simulink model "simulink_course_proj"  (R2026a)
settings: Solver=VariableStepAuto  StopTime=2
libraries: slpidlib x1
settings Model: Creator=noahhansen  LastModifiedBy=noahhansen

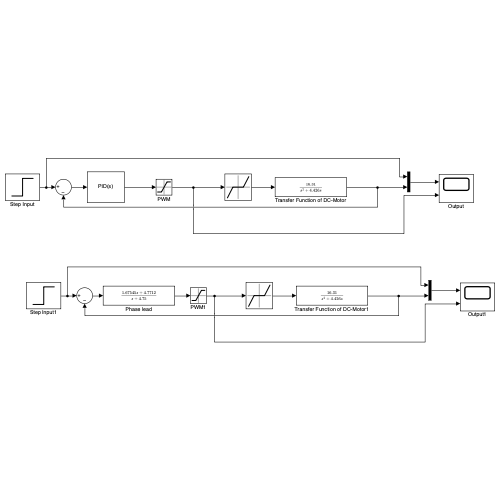
[thumbnail: Simulink's stored preview of the top-level diagram]
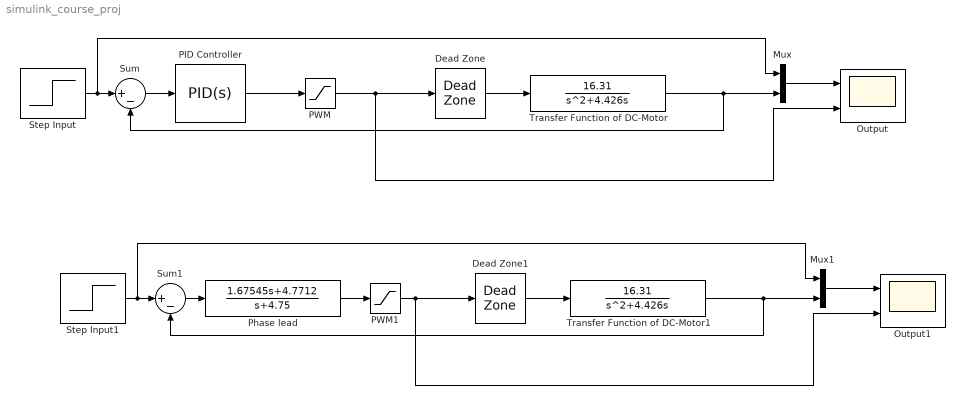
== system simulink_course_proj ==
  Dead Zone : DeadZone  LowerValue=-40  UpperValue=40
  Dead Zone1 : DeadZone  LowerValue=-40  UpperValue=40
  Mux : Mux  Inputs=2
  Mux1 : Mux  Inputs=2
  Output : Scope  NumInputPorts=2
      settings: TimeDisplayOffset=-0.1  ActiveDisplayYMinimum=-2  ActiveDisplayYMaximum=25  YLabel=Angle (degrees)
  Output1 : Scope  NumInputPorts=2
      settings: TimeDisplayOffset=-0.1  ActiveDisplayYMinimum=-10.6993  ActiveDisplayYMaximum=40  YLabel=Angle (degrees)
  PID Controller : slpidlib/PID Controller  Controller=PID  Form=Parallel  TimeDomain=Continuous-time  UseExternalTs=off  SampleTime=-1  IntegratorMethod=Forward Euler  FilterMethod=Forward Euler  ControllerParametersSource=internal  P=29  I=5  UseKiTs=off  D=1.4  UseExternalDerivativeSource=off  N=100  UseFilter=on  TunerSelectOption=Transfer Function Based (PID Tuner App)  InitialConditionSource=internal  InitialConditionForIntegrator=0  InitialConditionForFilter=0  DifferentiatorICPrevScaledInput=0  ExternalReset=none  TrackingMode=off  Kt=1  LimitOutput=off  SatLimitsSource=internal  UpperSaturationLimit=inf  LowerSaturationLimit=-inf  LinearizeAsGain=on  AntiWindupMode=none  Kb=1  LimitIntegrator=off  UpperIntegratorSaturationLimit=inf  LowerIntegratorSaturationLimit=-inf  POutMin=[]  POutMax=[]  IOutMin=[]  IOutMax=[]  DOutMin=[]  DOutMax=[]  NOutMin=[]  NOutMax=[]  SumOutMin=[]  SumOutMax=[]  SaturationOutMin=[]  SaturationOutMax=[]  PParamMin=[]  PParamMax=[]  IParamMin=[]  IParamMax=[]  DParamMin=[]  DParamMax=[]  NParamMin=[]  NParamMax=[]  KbParamMin=[]  KbParamMax=[]  KtParamMin=[]  KtParamMax=[]  KbOutMin=[]  KbOutMax=[]  KtOutMin=[]  KtOutMax=[]  IntegratorOutMin=[]  IntegratorOutMax=[]  FilterOutMin=[]  FilterOutMax=[]  SumI1OutMin=[]  SumI1OutMax=[]  SumI2OutMin=[]  SumI2OutMax=[]  SumI3OutMin=[]  SumI3OutMax=[]  SumI4OutMin=[]  SumI4OutMax=[]  SumDOutMin=[]  SumDOutMax=[]  DifferentiatorOutMin=[]  DifferentiatorOutMax=[]  FilterDiffOutCoefMin=[]  FilterDiffOutCoefMax=[]  ReciprocalOutMin=[]  ReciprocalOutMax=[]  SumDenOutMin=[]  SumDenOutMax=[]  SumNumOutMin=[]  SumNumOutMax=[]  DivideOutMin=[]  DivideOutMax=[]  UdiffTsProdOutMin=[]  UdiffTsProdOutMax=[]  NTsProdOutMin=[]  NTsProdOutMax=[]  UintegralTsProdOutMin=[]  UintegralTsProdOutMax=[]  UngainTsProdOutMin=[]  UngainTsProdOutMax=[]  ClampingZeroOutDataTypeStr=Inherit: Inherit via back propagation  ClampingZeroOutMin=[]  ClampingZeroOutMax=[]  FilterDenConstantOutDataTypeStr=Inherit: Inherit via back propagation  FilterDenConstantOutMin=[]  FilterDenConstantOutMax=[]  PCopyOutDataTypeStr=Inherit: Inherit via back propagation  PCopyOutMin=[]  PCopyOutMax=[]  NCopyOutDataTypeStr=Inherit: Inherit via back propagation  NCopyOutMin=[]  NCopyOutMax=[]  IntegratorContinuousStateAttributes=''  IntegratorStateMustResolveToSignalObject=off  IntegratorRTWStateStorageClass=Auto  FilterContinuousStateAttributes=''  FilterStateMustResolveToSignalObject=off  FilterRTWStateStorageClass=Auto  ParallelPVariant=InternalParameters  IdealPVariant=Disabled  IVariant=InternalParameters  DVariant=InternalParameters  IntegratorVariant=Continuous  SatVariant=Disabled  AWVariant=Passthrough  PCopyVariant=Disabled  TRVariant=Disabled  FdbkBlocksVariant=Forward  IdealPFdbkVariant=Disabled  SatFdbkVariant=Disabled  DerivativeFilterVariant=ContFilter  NVariant=InternalParameters  NCopyVariant=Disabled  FilterICVariant=InternalICsFilter  IntegratorICVariant=InternalICs  ExternalResetVariant=Disabled  TRSumVariant=Passthrough  SumFdbkVariant=Disabled  SumVariant=Sum_PID  TsampFilterVariant=InternalTs  TsampNgainVariant=Passthrough  TsampIntegralVariant=Passthrough  ExternalSaturationOutDataTypeStr=Inherit: Same as second input  DerivativeSourceVariant=ErrorSignal  PreIntVariant=InternalPreInt
  PWM : Saturate  UpperLimit=255  LowerLimit=-255
  PWM1 : Saturate  UpperLimit=255  LowerLimit=-255
  Phase lead : TransferFcn  Numerator=[1.67545 4.7712]  Denominator=[1 4.75]
  Step Input : Step  Time=0.1  FinalValue=20  SampleTime=0
  Step Input1 : Step  Time=0.1  FinalValue=30  SampleTime=0
  Sum : Sum  Inputs=|+-
  Sum1 : Sum  Inputs=|+-
  Transfer Function of DC-Motor : TransferFcn  Numerator=[16.31]  Denominator=[1 4.426 0]
  Transfer Function of DC-Motor1 : TransferFcn  Numerator=[16.31]  Denominator=[1 4.426 0]
  wires:
  Transfer Function of DC-Motor/1 -> Mux/2, Sum/2
  Mux/1 -> Output/1
  PID Controller/1 -> PWM/1
  PWM/1 -> Output/2, Dead Zone/1
  Dead Zone/1 -> Transfer Function of DC-Motor/1
  Step Input/1 -> Sum/1, Mux/1
  Sum/1 -> PID Controller/1
  PWM1/1 -> Output1/2, Dead Zone1/1
  Mux1/1 -> Output1/1
  Transfer Function of DC-Motor1/1 -> Mux1/2, Sum1/2
  Step Input1/1 -> Sum1/1, Mux1/1
  Dead Zone1/1 -> Transfer Function of DC-Motor1/1
  Phase lead/1 -> PWM1/1
  Sum1/1 -> Phase lead/1
